simulink model "compliment"  (R2016a)
settings: Solver=VariableStepAuto  StartTime=0.0  StopTime=10.0  RelTol=1e-3
libraries: visionsources x2, visionconversions x1
settings Model: Creator=Auroshis  LastModifiedBy=Auroshis

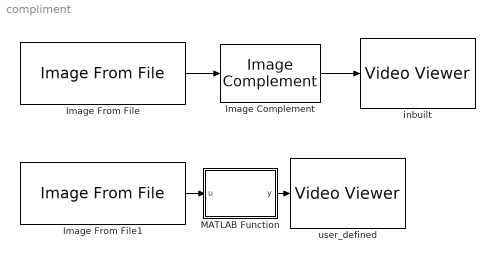
== system compliment ==
  Image Complement : visionconversions/Image Complement
  Image From File : visionsources/Image From File  Tag=vipblks_nd  FileName=cameraman.tif  imagePorts=One multidimensional signal  Ts=0.1  ImageDataType=Inherit from input image  Signed=on  WordLength=16  sdImageDataType=uint(8)  FractionLengthMode=User-defined  FractionLength=15  OutPortLabels=R|G|B
  Image From File1 : visionsources/Image From File  Tag=vipblks_nd  FileName=cameraman.tif  imagePorts=One multidimensional signal  Ts=0.1  ImageDataType=Inherit from input image  Signed=on  WordLength=16  sdImageDataType=uint(8)  FractionLengthMode=User-defined  FractionLength=15  OutPortLabels=R|G|B
  MATLAB Function : MATLAB Function  TreatAsAtomicUnit=on
  inbuilt : VideoViewer
  user_defined : VideoViewer  FigPos=[341 748.4 409.6 300]
  wires:
  Image From File/1 -> Image Complement/1
  Image Complement/1 -> inbuilt/1
  Image From File1/1 -> MATLAB Function/1(u)
  MATLAB Function/1(y) -> user_defined/1

== matlab function compliment/MATLAB Function ==
  data: u input; y output
function y = fcn(u)
y = 255-u;
